simulink subsystem "ActiveDifferential"  (R2023a)
settings: Solver=VariableStepAuto  StartTime=0.0  StopTime=10.0  RelTol=1e-3
libraries: autolibshareddiff x1
settings Model: Creator=The MathWorks, Inc.  LastModifiedBy=The MathWorks, Inc.

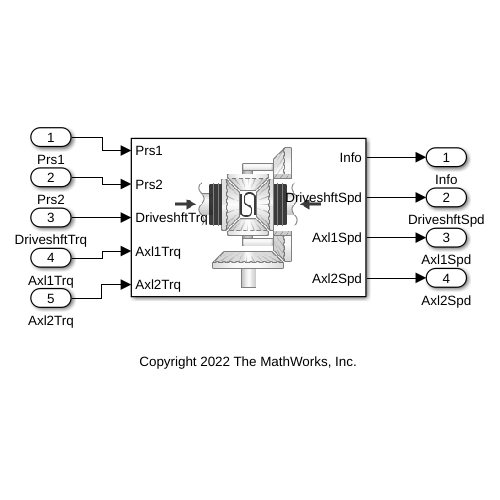
[thumbnail: Simulink's stored preview of the top-level diagram]
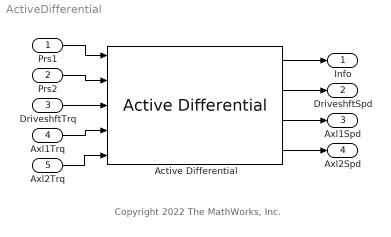
== system ActiveDifferential ==
  note: Copyright 2022 The MathWorks, Inc.
  Prs1 : Inport
  Prs2 : Inport  Port=2
  DriveshftTrq : Inport  Port=3
  Axl1Trq : Inport  Port=4
  Axl2Trq : Inport  Port=5
  Active Differential : autolibshareddiff/Active Differential  VariantControl=Active Differential  diffType=Spur gears, superposition clutches  Ns1=PlntDiffrntlCltch1CaseGearRatio  Ns2=PlntDiffrntlCltch2CaseGearRatio  Jgc=PlntDiffrntlThreeGangGearInertia  Np1=PlntDiffrntlCltchAxl1CarrGearRatio  Js1=PlntDiffrntlCltchAxl1SunGearInertia  Jc1=PlntDiffrntlCltchAxl1CarrInertia  Jr1=PlntDiffrntlCltchAxl1RingInertia  Np2=PlntDiffrntlCltchAxl2CarrGearRatio  Js2=PlntDiffrntlCltchAxl2SunGearInertia  Jc2=PlntDiffrntlCltchAxl2CarrInertia  Jr2=PlntDiffrntlCltchAxl2RingInertia  shaftSwitchMask=To the left of center-line  Ndiff=PlntDiffrntlRatio  Jd=PlntDiffrntlCarrInertia  bd=PlntDiffrntlCarrDamp  Jw1=PlntDiffrntlAxl1Inertia  bw1=PlntDiffrntlAxl1Damp  Jw2=PlntDiffrntlAxl2Inertia  bw2=PlntDiffrntlAxl2Damp  omegaw1o=PlntDiffrntlAxl1InitVel  omegaw2o=PlntDiffrntlAxl2InitVel  couplingType=Pre-loaded ideal clutch  Aeff=PlntDiffrntlCltchAppPrsArea  Ndisks=PlntDiffrntlCltchNumDisk  Reff=PlntDiffrntlCltchRadius  Fc=PlntDiffrntlCltchPreloadForce  muc=PlntDiffrntlCltchFricVect  dw=PlntDiffrntlCltchSpdVect  TdPdw=PlntDiffrntlCltchTrqSlipSpdVect  pT=PlntDiffrntlCltchPrsVect  dwT=PlntDiffrntlCltchSlipSpdVect  tauC=PlntDiffrntlCltchCplngTimeCnst  IdealInterpMethod=Linear point-slope  IdealExtrapMethod=Clip  TdwInterpMethod=Linear point-slope  TdwExtrapMethod=Clip  maxAbsSpd=5e3  aMode=6  blkID=0
  Info : Outport
  DriveshftSpd : Outport  Port=2
  Axl1Spd : Outport  Port=3
  Axl2Spd : Outport  Port=4
  wires:
  Active Differential/1 -> Info/1
  Active Differential/2 -> DriveshftSpd/1
  Active Differential/3 -> Axl1Spd/1
  Active Differential/4 -> Axl2Spd/1
  DriveshftTrq/1 -> Active Differential/3
  Axl2Trq/1 -> Active Differential/5
  Axl1Trq/1 -> Active Differential/4
  Prs2/1 -> Active Differential/2
  Prs1/1 -> Active Differential/1
